simulink model "simuConvectidorCD_CD"  (R2022b)
settings: Solver=VariableStepAuto  StartTime=0.0  StopTime=.01  MaxStep=.0001  RelTol=1e-3
values from neighbouring files (symbols this model uses):
  C = .00001    (= 1e-05)    [matlabConverrtidorCD_CD.m]    (also in scriptSimuConvertidorCD_CD.m)
  frecuencia = 100000    [matlabConverrtidorCD_CD.m]    (also in scriptSimuConvertidorCD_CD.m)
  L = .002    (= 0.002)    [matlabConverrtidorCD_CD.m]    (also in scriptSimuConvertidorCD_CD.m)
  PWM = zeros(length(time),1)    [matlabConverrtidorCD_CD.m]    (also in scriptSimuConvertidorCD_CD.m = 0.4)
  R = 10    [matlabConverrtidorCD_CD.m]    (also in scriptSimuConvertidorCD_CD.m)
  Uin = 32    [matlabConverrtidorCD_CD.m]    (also in scriptSimuConvertidorCD_CD.m)
libraries: simulink x1
settings Model: Creator=frayg  LastModifiedBy=frayg

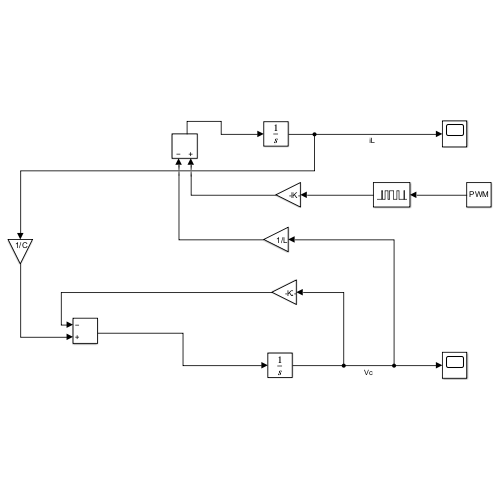
[thumbnail: Simulink's stored preview of the top-level diagram]
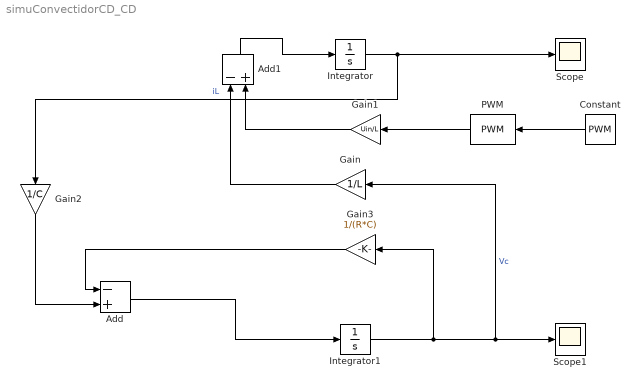
== system simuConvectidorCD_CD ==
  Add : Sum  Inputs=-+
  Add1 : Sum  Inputs=-+
  Constant : Constant  Value=PWM
  Gain : Gain  Gain=1/L
  Gain1 : Gain  Gain=Uin/L
  Gain2 : Gain  Gain=1/C
  Gain3 : Gain  Gain=1/(R*C)
  Integrator : Integrator
  Integrator1 : Integrator
  PWM : simulink/Discontinuities/PWM  DisableCoverage=on  Period=1/frecuencia  InitialDelay=0  DisallowZeroDutyCycle=off  RunAtFixedTimeIntervals=on  SampleTime=1/(frecuencia*5)
  Scope : Scope
  Scope1 : Scope
  wires:
  Integrator/1 -> Scope/1, Gain2/1  "iL"
  Integrator1/1 -> Gain3/1, Scope1/1, Gain/1  "Vc"
  Gain/1 -> Add1/1
  Gain1/1 -> Add1/2
  Constant/1 -> PWM/1
  PWM/1 -> Gain1/1
  Add/1 -> Integrator1/1
  Gain2/1 -> Add/2
  Gain3/1 -> Add/1
  Add1/1 -> Integrator/1
